simulink model "Observer"  (R2018b)
settings: Solver=FixedStepAuto  StartTime=0.0  StopTime=2  RelTol=1e-3
undefined symbols (not defined in the file or in its folder): A, B, C, D
libraries: dspstat3 x1, peLuenbergerObserver x1, simulink x1, pePwmGenerator x1, powerlib_meascontrol x1
settings Model: Creator=Roberto  LastModifiedBy=Roberto

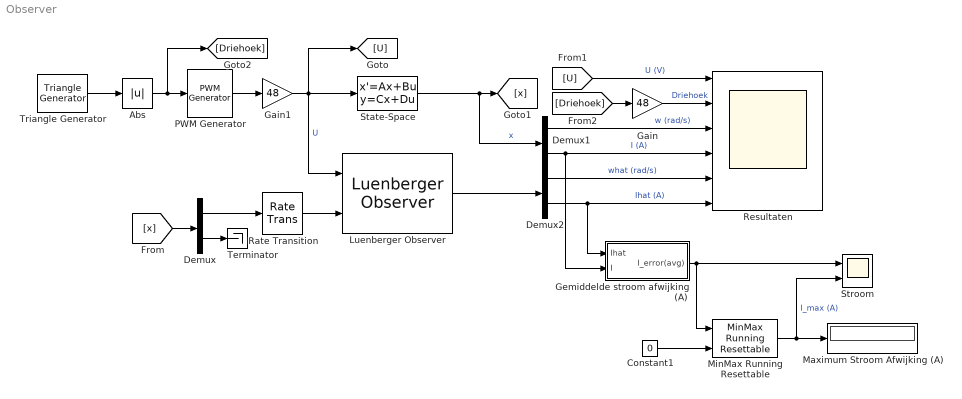
== system Observer ==
  Abs : Abs
  Constant1 : Constant  Value=0
  Demux : Demux  Outputs=2
  Demux1 : Demux  Outputs=2
  Demux2 : Demux  Outputs=2
  Gain : Gain  Gain=48
  Gain1 : Gain  Gain=48
  Gemiddelde stroom afwijking (A) : Subsystem
  Luenberger Observer : peLuenbergerObserver/Luenberger Observer  StateSpaceType=Continuous-time  Ad=Adh  Bd=Bdh  Cd=C  Dd=0  A=A  B=B  C=C  D=D  ObserverDesign=Observer gain  Ld=L  DesiredEigenvalues=eigenVal  x0=[0 0]  Tsd=0.1  Ts=1e-6
  Maximum Stroom Afwijking (A) : Display
  MinMax Running Resettable : simulink/Math Operations/MinMax Running Resettable  Function=max  vinit=0.0
  PWM Generator : pePwmGenerator/PWM Generator  CarrCount=Up  Tper=1/20000  Ts=1e-6
  Rate Transition : RateTransition  OutPortSampleTime=1/100000
  Resultaten : Scope  NumInputPorts=6
  State-Space : StateSpace  A=A  B=B  C=eye(2)  D=[0; 0]  InitialCondition=0
  Stroom : Scope  NumInputPorts=2
  Terminator : Terminator
  Triangle Generator : powerlib_meascontrol/Pulse & Signal Generators/Triangle Generator  Freq=0.5  Phase=90  Ts=1e-6
  wires:
  State-Space/1 -> [x], Demux1/1  "x"
  Demux1/1 -> Resultaten/3  "w (rad/s)"
  Demux2/1 -> Resultaten/5  "what (rad/s)"
  Demux1/2 -> Resultaten/4, Gemiddelde stroom afwijking (A)/2(I)  "I (A)"
  Demux2/2 -> Gemiddelde stroom afwijking (A)/1(Ihat), Resultaten/6  "Ihat (A)"
  Luenberger Observer/1 -> Demux2/1
  Demux/1 -> Rate Transition/1
  PWM Generator/1 -> Gain1/1
  Abs/1 -> [Driehoek], PWM Generator/1
  Gain1/1 -> Luenberger Observer/1, [U], State-Space/1  "U"
  Rate Transition/1 -> Luenberger Observer/2
  Triangle Generator/1 -> Abs/1
  [x] -> Demux/1
  Demux/2 -> Terminator/1
  [U] -> Resultaten/1  "U (V)"
  Gemiddelde stroom afwijking (A)/1(I_error(avg)) -> Stroom/1, MinMax Running Resettable/1
  [Driehoek] -> Gain/1
  Gain/1 -> Resultaten/2  "Driehoek"
  Constant1/1 -> MinMax Running Resettable/2
  MinMax Running Resettable/1 -> Stroom/2, Maximum Stroom Afwijking (A)/1  "I_max (A)"

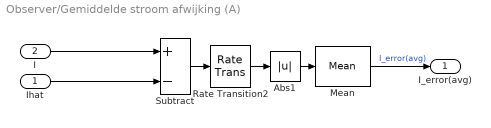
== system Observer/Gemiddelde stroom afwijking (A) ==
  Ihat : Inport
  I : Inport  Port=2
  Abs1 : Abs
  Mean : dspstat3/Mean  run=on  reset_popup=None  directionMode=Entire input  dimension=1  roiEnable=off  roiType=Rectangles  roiPortion=Entire ROI  roiOutput=Individual statistics for each ROI  roiFlag=off  roundingMode=Floor  overflowMode=off  outputDataTypeStr=Inherit: Same as accumulator  outputMin=[]  outputMax=[]  outputLastDataTypeStr=Inherit: Same as accumulator
  Rate Transition2 : RateTransition  OutPortSampleTime=1e-6
  Subtract : Sum  Inputs=+-
  I_error(avg) : Outport
  wires:
  I/1 -> Subtract/1
  Abs1/1 -> Mean/1
  Subtract/1 -> Rate Transition2/1
  Rate Transition2/1 -> Abs1/1
  Mean/1 -> I_error(avg)/1  "I_error(avg)"
  Ihat/1 -> Subtract/2
